simulink model "math_comparison"  (R2021a)
settings: Solver=VariableStepAuto  StartTime=0.0  StopTime=800  RelTol=1e-3
values from neighbouring files (symbols this model uses):
  A = [-0.0299243213669892 0.0256028069981396 ... (first row only)    [m3007.m]    (also in process_parameters.m = [-1/Tv, 0, 0; real_data_2.m = [-1/Tv, 0, 0; rls_algorithm.m = [-1/Tv, 0, 0)
  A1 = 450    [process_parameters.m]    (also in real_data_2.m; rls_algorithm.m)
  B = [0.00171378115848002; 0]    [m3007.m]    (also in process_parameters.m = [Kv/Tv; 0; 0]; real_data_2.m = [Kv/Tv; 0; 0]; rls_algorithm.m = [Kv/Tv; 0; 0])
  C = [0, 1]    [m3007.m]    (also in process_parameters.m = [0, 0, 1]; real_data_2.m = [0, 0, 1]; rls_algorithm.m = [0, 0, 1])
  g = 981    [process_parameters.m]    (also in real_data_2.m; rls_algorithm.m)
  h10 = data.WaterLevelTank1(start_index)    [m3007.m]    (also in process_parameters.m = 4.69; real_data_2.m = 4.69; rls_algorithm.m = 4.69)
  h20 = data.WaterLevelTank2(start_index)    [m3007.m]    (also in process_parameters.m = 3.39; real_data_2.m = 3.39; rls_algorithm.m = 3.39)
  K12A = K3*A1/sqrt(2*g)    [process_parameters.m]    (also in real_data_2.m; rls_algorithm.m)
  K12B = K2*A1/sqrt(2*g)    [process_parameters.m]    (also in real_data_2.m; rls_algorithm.m)
  K1d = K4*A1/sqrt(2*g)    [process_parameters.m]    (also in real_data_2.m; rls_algorithm.m)
  K2d = K4*A1/sqrt(2*g)    [process_parameters.m]    (also in real_data_2.m; rls_algorithm.m)
  Ki = K1*A1/sqrt(2*g)    [process_parameters.m]    (also in real_data_2.m; rls_algorithm.m)
  Kv = 3.0519 + 0.3    (= 3.3519)    [process_parameters.m]    (also in real_data_2.m = 3.2519; rls_algorithm.m = 3.2519)
  qu0 = data.InletFlow(start_index)*(1000/60)    [m3007.m]    (also in process_parameters.m = 93; real_data_2.m = 82; rls_algorithm.m = 82)
  Ts = 0.1    [process_parameters.m]    (also in real_data_2.m = 0.01; rls_algorithm.m)
  Tv = 1.74    [process_parameters.m]    (also in real_data_2.m; rls_algorithm.m)
settings Model: Creator=matij  LastModifiedBy=matij

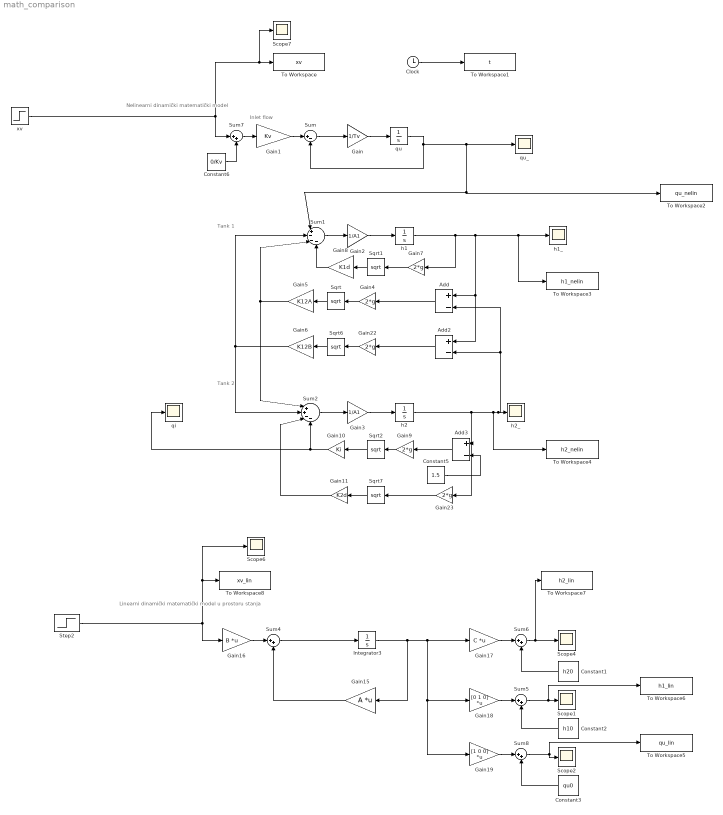
== system math_comparison ==
  note: Tank 2
  note: Tank 1
  note: Nelinearni dinamički matematički model
  note: Inlet flow
  note: Linearni dinamički matematički model u prostoru stanja
  Add : Sum  Inputs=+-
  Add2 : Sum  Inputs=+-
  Add3 : Sum  Inputs=+-
  Clock : Clock
  Constant1 : Constant  Value=h20
  Constant2 : Constant  Value=h10
  Constant3 : Constant  Value=qu0
  Constant5 : Constant  Value=1.5
  Constant6 : Constant  Value=0/Kv
  Gain : Gain  Gain=1/Tv
  Gain1 : Gain  Gain=Kv
  Gain10 : Gain  Gain=Ki
  Gain11 : Gain  Gain=K2d
  Gain15 : Gain  Gain=A  Multiplication=Matrix(K*u)
  Gain16 : Gain  Gain=B  Multiplication=Matrix(K*u)
  Gain17 : Gain  Gain=C  Multiplication=Matrix(K*u)
  Gain18 : Gain  Gain=[0 1 0]  Multiplication=Matrix(K*u)
  Gain19 : Gain  Gain=[1 0 0]  Multiplication=Matrix(K*u)
  Gain2 : Gain  Gain=1/A1
  Gain{4,7,9,22..23} (5 alike) : Gain  Gain=2*g
  Gain3 : Gain  Gain=1/A1
  Gain5 : Gain  Gain=K12A
  Gain6 : Gain  Gain=K12B
  Gain8 : Gain  Gain=K1d
  Integrator3 : Integrator
  Scope{1..2,4,6..7} (5 alike) : Scope
  Sqrt{,1..2,6..7} (5 alike) : Sqrt  SaturateOnIntegerOverflow=on
  Step2 : Step  Time=0  After=20  SampleTime=0
  Sum : Sum  Inputs=|+-
  Sum1 : Sum  Inputs=|+---
  Sum2 : Sum  Inputs=|++--
  Sum{4..8} (5 alike) : Sum  Inputs=|++
  To Workspace : ToWorkspace  VariableName=xv  SampleTime=Ts
  To Workspace1 : ToWorkspace  VariableName=t  SampleTime=Ts
  To Workspace2 : ToWorkspace  VariableName=qu_nelin  SampleTime=Ts
  To Workspace3 : ToWorkspace  VariableName=h1_nelin  SampleTime=Ts
  To Workspace4 : ToWorkspace  VariableName=h2_nelin  SampleTime=Ts
  To Workspace5 : ToWorkspace  VariableName=qu_lin  SampleTime=Ts
  To Workspace6 : ToWorkspace  VariableName=h1_lin  SampleTime=Ts
  To Workspace7 : ToWorkspace  VariableName=h2_lin  SampleTime=Ts
  To Workspace8 : ToWorkspace  VariableName=xv_lin  SampleTime=Ts
  h1 : Integrator  InitialCondition=h10
  h1_ : Scope
  h2 : Integrator  InitialCondition=h20
  h2_ : Scope
  qi : Scope
  qu : Integrator  InitialCondition=qu0
  qu_ : Scope
  xv : Step  Time=0  Before=25  After=45  SampleTime=0
  wires:
  Gain19/1 -> Sum8/1
  Gain18/1 -> Sum5/1
  Constant5/1 -> Add3/2
  Integrator3/1 -> Gain17/1, Gain18/1, Gain19/1, Gain15/1
  Sum8/1 -> To Workspace5/1, Scope2/1
  Constant3/1 -> Sum8/2
  Sum6/1 -> To Workspace7/1, Scope4/1
  Constant2/1 -> Sum5/2
  Sum5/1 -> To Workspace6/1, Scope1/1
  Sum4/1 -> Integrator3/1
  Constant1/1 -> Sum6/2
  Sqrt6/1 -> Gain6/1
  Gain11/1 -> Sum2/3
  Gain5/1 -> Sum1/3, Sum2/1
  Sum7/1 -> Gain1/1
  Step2/1 -> Gain16/1, Scope6/1, To Workspace8/1
  Gain8/1 -> Sum1/4
  Sum/1 -> Gain/1
  Gain16/1 -> Sum4/1
  Add3/1 -> Gain9/1
  Gain1/1 -> Sum/1
  Add/1 -> Gain4/1
  Gain10/1 -> qi/1, Sum2/4
  Gain2/1 -> h1/1
  xv/1 -> Sum7/1, To Workspace/1, Scope7/1
  Gain3/1 -> h2/1
  Sum2/1 -> Gain3/1
  Gain23/1 -> Sqrt7/1
  qu/1 -> Sum1/1, To Workspace2/1, qu_/1, Sum/2
  Gain4/1 -> Sqrt/1
  Gain7/1 -> Sqrt1/1
  Constant6/1 -> Sum7/2
  Gain6/1 -> Sum1/2, Sum2/2
  h1/1 -> Add2/1, Add/1, To Workspace3/1, h1_/1, Gain7/1
  Sqrt7/1 -> Gain11/1
  Sqrt2/1 -> Gain10/1
  Gain22/1 -> Sqrt6/1
  Sqrt/1 -> Gain5/1
  Add2/1 -> Gain22/1
  Sum1/1 -> Gain2/1
  Clock/1 -> To Workspace1/1
  h2/1 -> Gain23/1, Add3/1, Add/2, Add2/2, h2_/1, To Workspace4/1
  Gain9/1 -> Sqrt2/1
  Gain15/1 -> Sum4/2
  Sqrt1/1 -> Gain8/1
  Gain17/1 -> Sum6/1
  Gain/1 -> qu/1
